simulink model "inversor_corrente_digital_analogicob"  (R2018a)
settings: Solver=ode45  StartTime=0.0  StopTime=0.1  MaxStep=1e-7  RelTol=1e-3  EnableMultiTasking=on
libraries: powerlib x14, powerlib_meascontrol x1
settings Model: Creator=Vilela  LastModifiedBy=Bruna Resende
settings DataIOCC: LimitDataPoints=on  SaveFormat=Array
settings OptimizationCC: LifeSpan=inf
settings DebuggingCC: UnderspecifiedInitializationDetection=Classic  MergeDetectMultiDrivingBlocksExec=none  SolverPrmCheckMsg=warning  StateNameClashWarn=warning  SFUnexpectedBacktrackingDiag=warning  SFNoUnconditionalDefaultTransitionDiag=warning  SFExecutionAtInitializationDiag=none
settings HardwareCC: ProdBitPerPointer=32  ProdBitPerSizeT=32  ProdBitPerPtrDiffT=32  ProdLargestAtomicFloat=None  ProdIntDivRoundTo=Undefined  ProdEndianess=Unspecified  ProdWordSize=32  ProdHWDeviceType=32-bit Generic
settings ModelReferenceCC: PropagateSignalLabelsOutOfModel=off
settings CodeAppCC: StateflowObjectComments=on
settings GRTTargetCC: TargetLangStandard=C89/C90 (ANSI)  GeneratePreprocessorConditionals=Disable all
settings ConfigComp: CovMetricSettings=dw  CovHtmlReporting=on  CovSaveCumulativeToWorkspaceVar=on  CovSaveSingleToWorkspaceVar=on  CovExternalEMLEnable=off

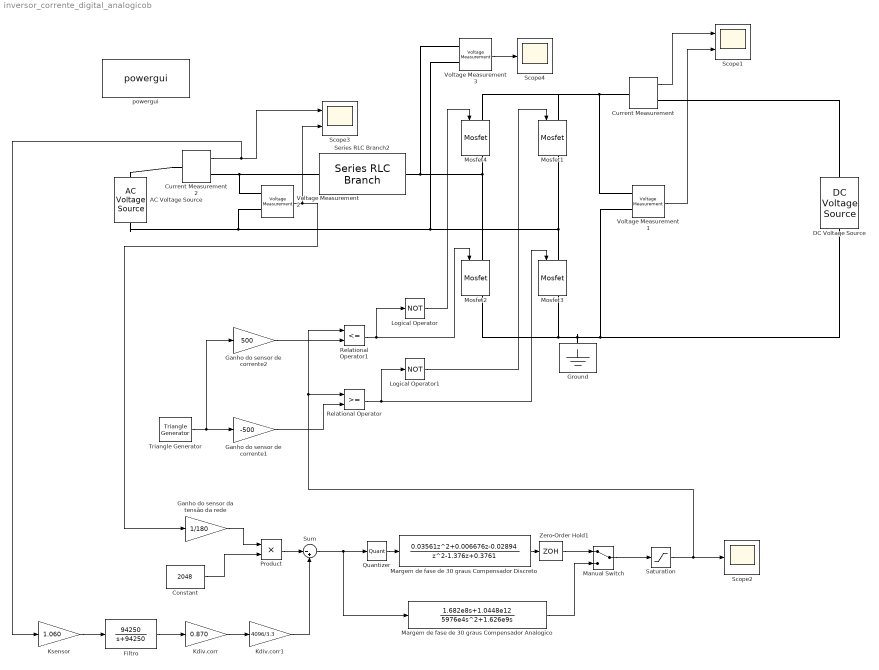
== system inversor_corrente_digital_analogicob ==
  AC Voltage Source : powerlib/Electrical Sources/AC Voltage Source  Amplitude=127*sqrt(2)  Phase=0  Frequency=60  SampleTime=0  Measurements=None  BusType=swing  Pref=10e3  Qref=0  Qmin=-inf  Qmax=+inf
  Constant : Constant  Value=2048
  Current Measurement : powerlib/Measurements/Current Measurement  PhasorSimulation=off  OutputType=Complex  PSBequivalent=0
  Current Measurement2 : powerlib/Measurements/Current Measurement  PhasorSimulation=off  OutputType=Complex  PSBequivalent=0
  DC Voltage Source : powerlib/Electrical Sources/DC Voltage Source  Amplitude=235  Measurements=None
  Filtro : TransferFcn  Numerator=[94250]  Denominator="[1  94250]"
  Ganho do sensor da tensão da rede : Gain  Gain=1/180
  Ganho do sensor de corrente1 : Gain  Gain=-500
  Ganho do sensor de corrente2 : Gain  Gain=500
  Ground : powerlib/Elements/Ground  LConnTagsString=a
  Kdiv.corr : Gain  Gain=0.870
  Kdiv.corr1 : Gain  Gain=4096/3.3
  Ksensor : Gain  Gain=1.060
  Logical Operator : Logic  Operator=NOT  AllPortsSameDT=off  OutDataTypeStr=boolean
  Logical Operator1 : Logic  Operator=NOT  AllPortsSameDT=off  OutDataTypeStr=boolean
  Manual Switch : ManualSwitch
  Margem de fase de 30 graus Compensador Analogico : TransferFcn  Numerator="[1.682e8  1.0448e12]"  Denominator="[5976e4  1.626e9   0 ]"
  Margem de fase de 30 graus Compensador Discreto : DiscreteTransferFcn  Numerator=[0.03561 0.006676 -0.02894]  Denominator=[1 -1.376 0.3761]  SampleTime=0.0000333333
  Mosfet{1..4} (4 alike) : powerlib/Power Electronics/Mosfet  Ron=0.1  Lon=0  Rd=0.01  Vfd=0  IC=0  Rs=1e5  Cs=inf  Measurements=on
  Product : Product
  Quantizer : Quantizer  QuantizationInterval=3/1024  SampleTime=0.0000333333
  Relational Operator : RelationalOperator  OutDataTypeStr=boolean  RndMeth=Nearest
  Relational Operator1 : RelationalOperator  Operator=<=  OutDataTypeStr=boolean  RndMeth=Nearest
  Saturation : Saturate  UpperLimit=480  LowerLimit=-480
  Scope1 : Scope  NumInputPorts=2
  Scope2 : Scope
  Scope3 : Scope  NumInputPorts=2
  Scope4 : Scope
  Series RLC Branch2 : powerlib/Elements/Series RLC Branch  LConnTagsString=__new0  RConnTagsString=__new0  BranchType=L  Resistance=10  Inductance=2.2e-3  SetiL0=off  InitialCurrent=0  Capacitance=100e-6  Setx0=off  InitialVoltage=0  Measurements=None
  Sum : Sum  Inputs=|-+
  Triangle Generator : powerlib_meascontrol/Pulse & Signal Generators/Triangle Generator  Freq=50e3  Phase=0  Ts=0
  Voltage Measurement1 : powerlib/Measurements/Voltage Measurement  PhasorSimulation=off  OutputType=Complex  PSBequivalent=0
  Voltage Measurement2 : powerlib/Measurements/Voltage Measurement  PhasorSimulation=off  OutputType=Complex  PSBequivalent=0
  Voltage Measurement3 : powerlib/Measurements/Voltage Measurement  PhasorSimulation=off  OutputType=Complex  PSBequivalent=0
  Zero-Order Hold1 : ZeroOrderHold  SampleTime=0.0000333333
  powergui : powerlib/powergui  Priority=1  SimulationMode=Continuous  SolverType=Tustin  SampleTime=50e-6  frequency=60  SPID=off  DisableSnubberDevices=off  DisableRonSwitches=off  DisableVfSwitches=off  SwTol=0  DisplayEquations=off  Interpol=off  ExternalGateDelay=off  methode=off  Ts=0  FunctionMessages=off  echomessages=off  HookPort=off  EnableUseOfTLC=off  x0status=blocks  frequencyindice=0  Pbase=100e6  ErrMax=1e-4  Iterations=50  UnitsV=V  UnitsW=W  buscounter=0  RestoreLinks=warning  ResistiveCurrentMeasurement=off  Frange=[0:2:500]  Ylog=off  Xlog=on  ShowGrid=off  save=off  variable=ZData  structure=0  ZoomFFT=off  StartTime=0.0  cycles=1  DisplayStyle=1  fundamental=60  FreqAxis=off  MaxFrequency=1000  frequencyindicesteady=1  RmsSteady=1  display=off
  wires:
  Voltage Measurement1/1 -> Scope1/2
  Triangle Generator/1 -> Ganho do sensor de corrente2/1, Ganho do sensor de corrente1/1
  Ganho do sensor de corrente1/1 -> Relational Operator/2
  Ganho do sensor de corrente2/1 -> Relational Operator1/2
  Saturation/1 -> Scope2/1, Relational Operator/1, Relational Operator1/1
  Relational Operator/1 -> Logical Operator1/1, Mosfet3/1
  Relational Operator1/1 -> Logical Operator/1, Mosfet2/1
  Logical Operator1/1 -> Mosfet1/1
  Logical Operator/1 -> Mosfet4/1
  Voltage Measurement2/1 -> Scope3/2, Ganho do sensor da tensão da rede/1
  Ganho do sensor da tensão da rede/1 -> Product/1
  Constant/1 -> Product/2
  Product/1 -> Sum/1
  Ksensor/1 -> Filtro/1
  Current Measurement/1 -> Scope1/1
  Voltage Measurement3/1 -> Scope4/1
  Quantizer/1 -> Margem de fase de 30 graus Compensador Discreto/1
  Sum/1 -> Margem de fase de 30 graus Compensador Analogico/1, Quantizer/1
  Margem de fase de 30 graus Compensador Analogico/1 -> Manual Switch/2
  Margem de fase de 30 graus Compensador Discreto/1 -> Zero-Order Hold1/1
  Manual Switch/1 -> Saturation/1
  Current Measurement2/1 -> Ksensor/1, Scope3/1
  Filtro/1 -> Kdiv.corr/1
  Kdiv.corr/1 -> Kdiv.corr1/1
  Kdiv.corr1/1 -> Sum/2
  Zero-Order Hold1/1 -> Manual Switch/1
  connections:
  Series RLC Branch2/LConn1 -- Voltage Measurement3/LConn1 -- Mosfet2/LConn1 -- Mosfet4/RConn1
  Voltage Measurement2/LConn2 -- Voltage Measurement3/LConn2 -- Mosfet3/LConn1 -- Mosfet1/RConn1 -- AC Voltage Source/LConn1
  Mosfet4/LConn1 -- Mosfet1/LConn1 -- Current Measurement/LConn1 -- Voltage Measurement1/LConn1
  Voltage Measurement1/LConn2 -- Mosfet2/RConn1 -- Mosfet3/RConn1 -- Ground/LConn1 -- DC Voltage Source/LConn1
  Current Measurement2/RConn1 -- Series RLC Branch2/RConn1 -- Voltage Measurement2/LConn1
  Current Measurement/RConn1 -- DC Voltage Source/RConn1
  Current Measurement2/LConn1 -- AC Voltage Source/RConn1
